simulink model "second_order_inversion_algorithms"  (R2019b)
settings: Solver=VariableStepAuto  StartTime=0.0  StopTime=4  RelTol=1e-3
undefined symbols (not defined in the file or in its folder): DiscIntNeverNeededParam, q0, q0_dot, Tc
settings Model: Creator=swl782203812  LastModifiedBy=Administrator
settings DebuggingCC: ArithmeticOperatorsInVariantConditions=warning
settings SFSimCC: CustomCodeUndefinedFunction=UseInterfaceOnly

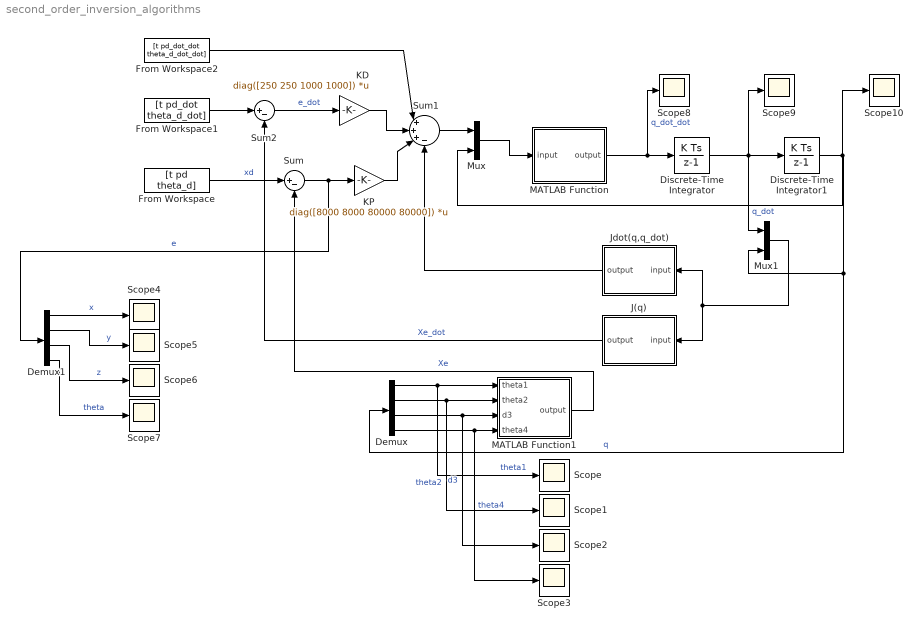
== system second_order_inversion_algorithms ==
  Demux : Demux
  Demux1 : Demux
  Discrete-Time Integrator : DiscreteIntegrator  InitialCondition=q0_dot  SampleTime=Tc  ICPrevOutput=DiscIntNeverNeededParam  ICPrevScaledInput=DiscIntNeverNeededParam
  Discrete-Time Integrator1 : DiscreteIntegrator  InitialCondition=q0  SampleTime=Tc  ICPrevOutput=DiscIntNeverNeededParam  ICPrevScaledInput=DiscIntNeverNeededParam
  From Workspace : FromWorkspace  VariableName=[t pd theta_d]  SampleTime=Tc
  From Workspace1 : FromWorkspace  VariableName=[t pd_dot theta_d_dot]  SampleTime=Tc
  From Workspace2 : FromWorkspace  VariableName=[t pd_dot_dot theta_d_dot_dot]  SampleTime=Tc
  J(q) : MATLAB Function  TreatAsAtomicUnit=on
  Jdot(q,q_dot) : MATLAB Function  TreatAsAtomicUnit=on
  KD : Gain  Gain=diag([250 250 1000 1000])  Multiplication=Matrix(K*u) (u vector)
  KP : Gain  Gain=diag([8000 8000 80000 80000])  Multiplication=Matrix(K*u) (u vector)
  MATLAB Function : MATLAB Function  TreatAsAtomicUnit=on
  MATLAB Function1 : MATLAB Function  TreatAsAtomicUnit=on
  Mux : Mux  Inputs=2
  Mux1 : Mux  Inputs=2
  Scope{,1..10} (11 alike) : Scope
  Sum : Sum  Inputs=|+-
  Sum1 : Sum  Inputs=|+++-
  Sum2 : Sum  Inputs=|+-
  wires:
  From Workspace/1 -> Sum/1  "xd"
  Sum/1 -> Demux1/1, KP/1  "e"
  Discrete-Time Integrator/1 -> Scope9/1, Mux1/1, Discrete-Time Integrator1/1  "q_dot"
  From Workspace1/1 -> Sum2/1
  KP/1 -> Sum1/3
  MATLAB Function1/1(output) -> Sum/2  "Xe"
  Demux/1 -> Scope/1, MATLAB Function1/1(theta1)  "theta1"
  Demux/2 -> Scope1/1, MATLAB Function1/2(theta2)  "theta2"
  Demux/3 -> Scope2/1, MATLAB Function1/3(d3)  "d3"
  Demux/4 -> Scope3/1, MATLAB Function1/4(theta4)  "theta4"
  MATLAB Function/1(output) -> Scope8/1, Discrete-Time Integrator/1  "q_dot_dot"
  Sum1/1 -> Mux/1
  Mux/1 -> MATLAB Function/1(input)
  From Workspace2/1 -> Sum1/1
  Sum2/1 -> KD/1  "e_dot"
  Discrete-Time Integrator1/1 -> Scope10/1, Mux/2, Demux/1, Mux1/2  "q"
  Jdot(q,q_dot)/1(output) -> Sum1/4
  J(q)/1(output) -> Sum2/2  "Xe_dot"
  Mux1/1 -> Jdot(q,q_dot)/1(input), J(q)/1(input)
  KD/1 -> Sum1/2
  Demux1/1 -> Scope4/1  "x"
  Demux1/2 -> Scope5/1  "y"
  Demux1/3 -> Scope6/1  "z"
  Demux1/4 -> Scope7/1  "theta"

== matlab function second_order_inversion_algorithms/MATLAB Function ==
  data: input input; output output
function output=Jacobian_inverse(input)
%INPUT is (theta1, theta2, d3, theta4,xd_dot_plus_Ke) 
theta1=input(5,:); d1=0; a1=0.5; alpha1=0; %parameter link1
theta2=input(6,:); d2=0; a2=0.5; alpha2=0; %parameter link2
theta3=0; d3=input(7,:); a3=0; alpha3=0;  %parameter link3
theta4=input(8,:); d4=0; a4=0; alpha4=0;  %parameter link4
    Jv = [-0.5*(sin(theta1)+sin(theta1+theta2)) -0.5*sin(theta1+theta2) 0 0;
          0.5*(cos(theta1)+cos(theta1+theta2)) 0.5*cos(theta1+theta2) 0 0;
          0 0 -1 0; 
          1 1 0 1;];
    output = inv(Jv)*input(1:4,:);
end

== matlab function second_order_inversion_algorithms/MATLAB Function1 ==
  data: output output; theta1 input; theta2 input; d3 input; theta4 input
function output = direct_kinematic(theta1,theta2,d3,theta4)
% Direct kinematics function of SCARA 
    A01 = [cos(theta1) -sin(theta1) 0 0.5.*cos(theta1);
           sin(theta1) cos(theta1) 0 0.5.*sin(theta1);
           0 0 1 0;
           0 0 0 1];
    A12 = [cos(theta2) -sin(theta2) 0 0.5.*cos(theta2);
           sin(theta2) cos(theta2) 0 0.5.*sin(theta2);
           0 0 1 0;
           0 0 0 1];
    A23 = [1 0 0 0;
           0 1 0 0;
           0 0 1 1-d3;
           0 0 0 1];
    A34 = [cos(theta4) -sin(theta4) 0 0;
           sin(theta4) cos(theta4) 0 0;
           0 0 1 0;
           0 0 0 1];
    A04 = A01*A12*A23*A34;
    P = [0.5*cos(theta1)+0.5*cos(theta1+theta2);0.5*sin(theta1)+0.5*sin(theta1+theta2);1-d3;(theta1+theta2+theta4)];
    output = P;
end

== matlab function second_order_inversion_algorithms/Jdot(q,q_dot) ==
  data: input input; output output
function output = Jacobian_dot(input)
% Part 1 Jacobian Differential: J(q)_dot
    theta1 = input(5,:);
    theta2 = input(6,:);
    theta1_dot = input(1,:);
    theta2_dot = input(2,:);
    Jv = [-0.5*(sin(theta1)+sin(theta1+theta2)) -0.5*sin(theta1+theta2) 0 0;
          0.5*(cos(theta1)+cos(theta1+theta2)) 0.5*cos(theta1+theta2) 0 0;
          0 0 -1 0;
          1 1 0 1;];
     Jd = [-0.5*(cos(theta1)*theta1_dot+cos(theta1+theta2)*(theta1_dot)) -0.5*cos(theta1+theta2)*(theta2_dot) 0 0;
           -0.5*(sin(theta1)*theta1_dot+sin(theta1+theta2)*(theta1_dot)) -0.5*sin(theta1+theta2)*(theta2_dot) 0 0;
           0 0 0 0;
           0 0 0 0;];
    q_dot = [input(1,:); input(2,:); input(3,:); input(4,:)];
    output = Jd*q_dot;
end

== matlab function second_order_inversion_algorithms/J(q) ==
  data: input input; output output
function output = Jacobian(input)
% Part 1 Jacobian: J(q)
    theta1 = input(5,:);
    theta2 = input(6,:);
    Jv = [-0.5*(sin(theta1)+sin(theta1+theta2)) -0.5*sin(theta1+theta2) 0 0; 0.5*(cos(theta1)+cos(theta1+theta2)) 0.5*cos(theta1+theta2) 0 0; 0 0 -1 0; 1 1 0 1;];
    q_dot = [input(1,:); input(2,:); input(3,:); input(4,:)];
    output = Jv*q_dot;
end
